simulink model "example_02"  (R2019b)
settings: Solver=VariableStepAuto  StartTime=0.0  StopTime=100  RelTol=1e-12
undefined symbols (not defined in the file or in its folder): zq
libraries: DQ_SR_LIB_SIM x2
settings Model: Creator=AurelianoRivolta  LastModifiedBy=AurelianoRivolta

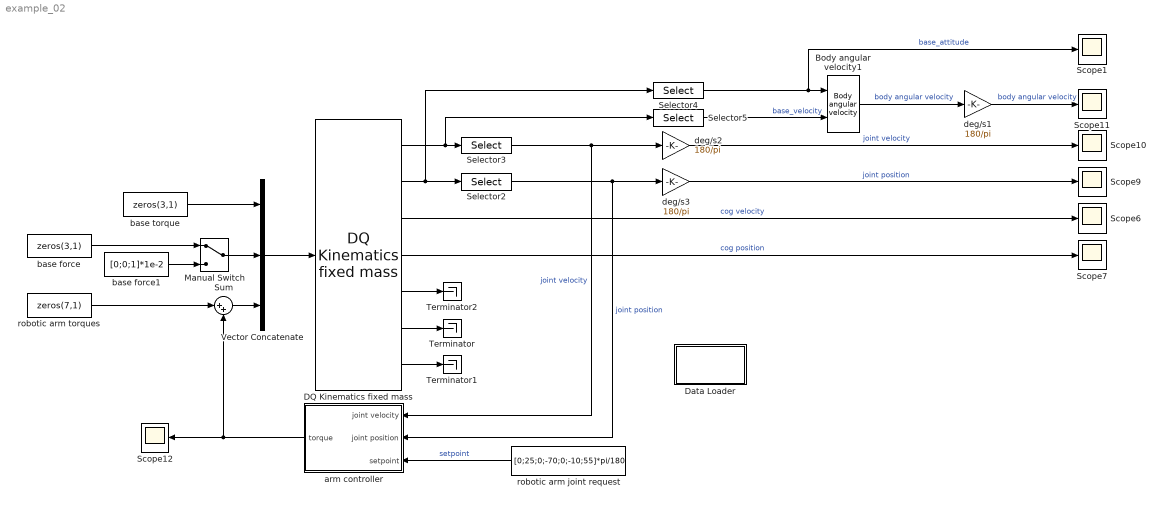
== system example_02 ==
  Body angular velocity1 : DQ_SR_LIB_SIM/Utilities/Body  angular velocity
  DQ Kinematics fixed mass : DQ_SR_LIB_SIM/DQ Kinematics fixed mass  dynfun='OR_sys_gen'  Gswitch=No gravity  n_bodies=2  n_var0=5  n_ext=7  q_norm_in=[1:4]'  NORMONOFF=on  II=II2  X0=[zeros(4,1);zeros(7,1)+randn(7,1)*0e-3;zq;zeros(7,1)]  XCG0=zeros(6,1)  UPPERSAT=Inf  LOWERSAT=-Inf
  Data Loader : Subsystem  InitFcn=|
      | [DIM,II2,endeff,end_eff_index,laserDQ,laserDQarm,cam_e_dq,cam_e_id,cam_l_dq,cam_r_dq,cam_lr_id,baseline,...
      | Mc,Nc,Oc,Kc,Gc,Ic,KV,KP,TV,DT_wakeup,PP,dPP,PM,THR]=chaser_robot_data
  Manual Switch : ManualSwitch
  Scope{1,6..7,9..12} (7 alike) : Scope
  Selector2 : Selector  InputPortWidth=11  IndexOptions=Index vector (dialog)  Indices=5:11  OutputSizes=1
  Selector3 : Selector  InputPortWidth=11  IndexOptions=Index vector (dialog)  Indices=5:11  OutputSizes=1
  Selector4 : Selector  InputPortWidth=11  IndexOptions=Index vector (dialog)  Indices=1:4  OutputSizes=1
  Selector5 : Selector  InputPortWidth=11  IndexOptions=Index vector (dialog)  Indices=1:4  OutputSizes=1
  Sum : Sum  Inputs=|++
  Terminator : Terminator
  Terminator1 : Terminator
  Terminator2 : Terminator
  Vector Concatenate : Concatenate  NumInputs=3
  arm controller : Subsystem
  base force : Constant  Value=zeros(3,1)  VectorParams1D=off
  base force1 : Constant  Value=[0;0;1]*1e-2  VectorParams1D=off
  base torque : Constant  Value=zeros(3,1)  VectorParams1D=off
  deg/s1 : Gain  Gain=180/pi
  deg/s2 : Gain  Gain=180/pi
  deg/s3 : Gain  Gain=180/pi
  robotic arm joint request : Constant  Value=[0;25;0;-70;0;-10;55]*pi/180  VectorParams1D=off
  robotic arm torques : Constant  Value=zeros(7,1)  VectorParams1D=off
  wires:
  Vector Concatenate/1 -> DQ Kinematics fixed mass/1
  base torque/1 -> Vector Concatenate/1
  Sum/1 -> Vector Concatenate/3
  DQ Kinematics fixed mass/4 -> Scope7/1  "cog position"
  DQ Kinematics fixed mass/3 -> Scope6/1  "cog velocity"
  DQ Kinematics fixed mass/2 -> Selector4/1, Selector2/1
  Selector2/1 -> arm controller/2(joint position), deg/s3/1  "joint position"
  DQ Kinematics fixed mass/1 -> Selector5/1, Selector3/1
  Selector3/1 -> arm controller/1(joint velocity), deg/s2/1  "joint velocity"
  DQ Kinematics fixed mass/6 -> Terminator/1
  DQ Kinematics fixed mass/7 -> Terminator1/1
  robotic arm torques/1 -> Sum/1
  Selector4/1 -> Scope1/1, Body angular velocity1/1  "base_attitude"
  Selector5/1 -> Body angular velocity1/2  "base_velocity"
  Body angular velocity1/1 -> deg/s1/1  "body angular velocity"
  deg/s1/1 -> Scope11/1  "body angular velocity"
  deg/s2/1 -> Scope10/1  "joint velocity"
  deg/s3/1 -> Scope9/1  "joint position"
  DQ Kinematics fixed mass/5 -> Terminator2/1
  base force/1 -> Manual Switch/1
  base force1/1 -> Manual Switch/2
  Manual Switch/1 -> Vector Concatenate/2
  arm controller/1("torque ") -> Scope12/1, Sum/2
  robotic arm joint request/1 -> arm controller/3(setpoint)  "setpoint"

== system example_02/Data Loader ==

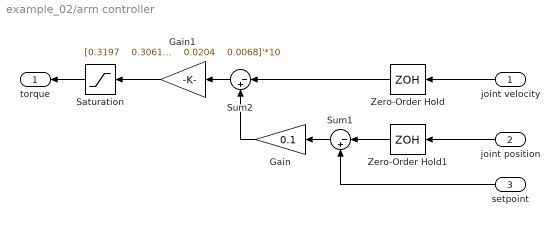
== system example_02/arm controller ==
  joint velocity : Inport
  joint position : Inport  Port=2
  setpoint : Inport  Port=3
  Gain : Gain  Gain=0.1
  Gain1 : Gain  Gain="[0.3197    0.3061    0.1701    0.1429    0.0340    0.0204    0.0068]'*10"
  Saturation : Saturate
  Sum1 : Sum  Inputs=|-+
  Sum2 : Sum  Inputs=|-+
  Zero-Order Hold : ZeroOrderHold  SampleTime=0.01
  Zero-Order Hold1 : ZeroOrderHold  SampleTime=0.01
  "torque " : Outport
  wires:
  Gain1/1 -> Saturation/1
  Gain/1 -> Sum2/2
  joint position/1 -> Zero-Order Hold1/1
  Zero-Order Hold1/1 -> Sum1/1
  Zero-Order Hold/1 -> Sum2/1
  setpoint/1 -> Sum1/2
  Sum2/1 -> Gain1/1
  Sum1/1 -> Gain/1
  Saturation/1 -> "torque "/1
  joint velocity/1 -> Zero-Order Hold/1
